simulink model "Simulink_FM"  (R2021b)
settings: Solver=VariableStepAuto  StartTime=0.0  StopTime=10  RelTol=1e-3
libraries: commanapbnd3 x2
settings Model: Creator=enrique  LastModifiedBy=enrique
settings SolverCC: AlgebraicLoopSolver=TrustRegion
settings DebuggingCC: SFMachineParentedDataDiag=warning

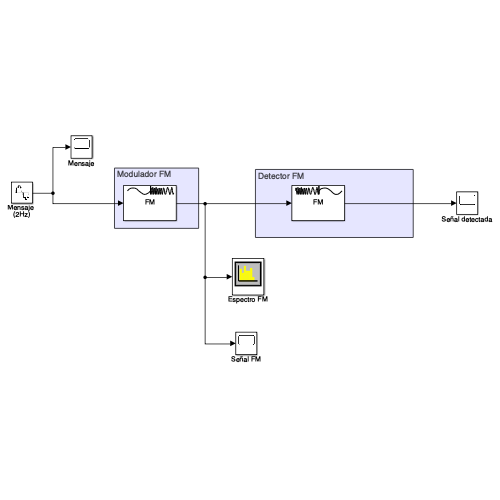
[thumbnail: Simulink's stored preview of the top-level diagram]
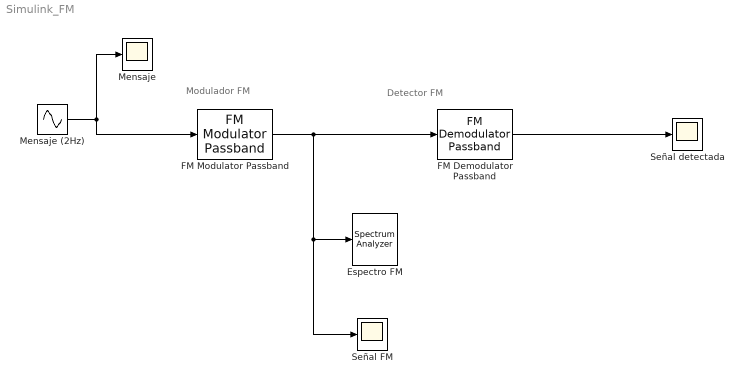
== system Simulink_FM ==
  note: Detector FM
  note: Modulador FM
  Espectro FM : SpectrumAnalyzer
  FM Demodulator Passband : commanapbnd3/FM Demodulator Passband  Fc=300  Ph=0  Kc=200  Ho=100
      settings: SourceProductBaseCode=CM
  FM Modulator Passband : commanapbnd3/FM Modulator Passband  Fc=300  Ph=0  Kc=200
      settings: SourceProductBaseCode=CM
  Mensaje : Scope
  "Mensaje (2Hz) " : Sin  Frequency=2*pi*2  SampleTime=1/5000
  Señal FM : Scope
  Señal detectada : Scope
  wires:
  "Mensaje (2Hz) "/1 -> FM Modulator Passband/1, Mensaje/1
  FM Modulator Passband/1 -> FM Demodulator Passband/1, Espectro FM/1, Señal FM/1
  FM Demodulator Passband/1 -> Señal detectada/1
